simulink model "QCar2_CameraDriving"  (R2025b)
settings: Solver=ode2  StartTime=0.0  StopTime=inf  FixedStep=1/100  RelTol=1e-3  EnableMultiTasking=on
InitFcn:
  | modelFile = get_param(bdroot,'FileName');
  | modelDir  = fileparts(modelFile);
  | 
  | addpath(modelDir); % so load_waypoints.m is found if it sits next to the model
  | addpath(fullfile(modelDir,".."));
  | 
  | wpFile = fullfile(modelDir, "waypoints.txt");
  | WP = load_waypoints(wpFile);
  | 
  | assignin("base","WP",WP);
model workspace (MAT data in the model file):
  camera_rate : Simulink.Parameter (value not decoded)
  depth_rate : Simulink.Parameter (value not decoded)
symbols that are objects in the model workspace (value not decoded): camera_rate, depth_rate
undefined symbols (not defined in the file or in its folder): gcbh, HIL, JPEG, Point, qc_get_step_size, Video3D, video_display_show
libraries: quarc_library x37, simulink x14
(part 3 of 3)

== matlab function QCar2_CameraDriving/obstacleDetection/Steering based image subselector ==
  data: pts output; depth input; region output; steering input
function [pts, region] = drawBox(depth, steering)
% Input: 640 x 360
mark = round(320 - (steering*260/0.5));
starting_index = mark+1-60;
region = double(depth(121:240, starting_index : starting_index + 119));
pts = [ 101, mark+1-60; 101, mark+60; 220, mark+60; 220, mark+1-60; 101, mark+1-60];
